simulink model "exampleTrackedSurface"  (Simulink 7.6)
settings: Solver=ode45  StartTime=180*24*3600  StopTime=190*24*3600  RelTol=1e-3
libraries: carnot x3
settings Model: Creator=drhf  LastModifiedBy=drhf
settings CodeAppCC: CustomSymbolStrType=$N$R$M_T

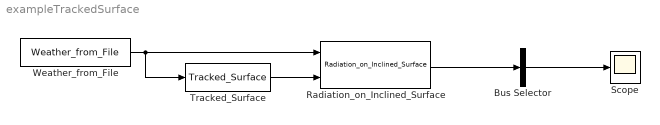
== system exampleTrackedSurface ==
  Bus Selector : BusSelector  OutputSignals=Solar_Radiation_direct_surface,Solar_Radiation_diffuse_surface  OutputAsBus=on
  Radiation_on_Inclined_Surface : carnot/Weather/Radiation_on_Inclined_Surface  SystemSampleTime=-1  sky=Perez 1990  reflect=0.2
  Scope : Scope
  Tracked_Surface : carnot/Weather/Tracked_Surface  SystemSampleTime=-1  tracktype=two axis tracking  inc=0  azi=0  rot=0  time=0
  Weather_from_File : carnot/Weather/Weather_from_File  SystemSampleTime=-1  file=DE_try13_avgYear  ext=.mat
  wires:
  Weather_from_File/1 -> Tracked_Surface/1, Radiation_on_Inclined_Surface/1
  Tracked_Surface/1 -> Radiation_on_Inclined_Surface/2
  Radiation_on_Inclined_Surface/1 -> Bus Selector/1
  Bus Selector/1 -> Scope/1
